simulink model "es2_sim2"  (R2023b)
settings: Solver=VariableStepAuto  StartTime=0.0  StopTime=10.0  RelTol=1e-3
values from neighbouring files (symbols this model uses):
  x0 = [3 5]'    [es2.m]    (also in es2_2.m = [3;5])
settings Model: Creator=stefa  LastModifiedBy=stefa

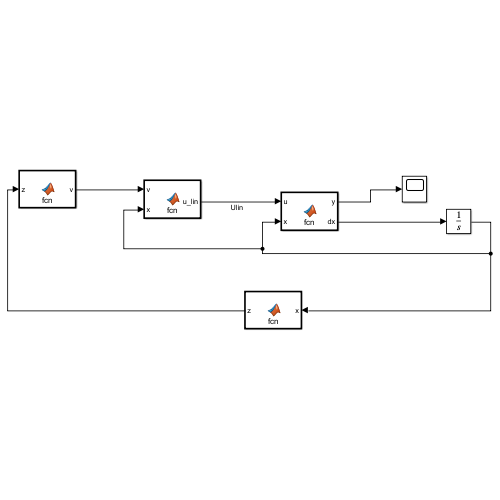
[thumbnail: Simulink's stored preview of the top-level diagram]
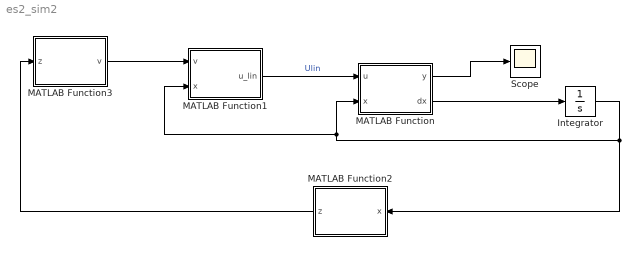
== system es2_sim2 ==
  Integrator : Integrator  InitialCondition=x0
  MATLAB Function : MATLAB Function  TreatAsAtomicUnit=on
  MATLAB Function1 : MATLAB Function  TreatAsAtomicUnit=on
  MATLAB Function2 : MATLAB Function  TreatAsAtomicUnit=on
  MATLAB Function3 : MATLAB Function  TreatAsAtomicUnit=on
  Scope : Scope
  wires:
  MATLAB Function/1(y) -> Scope/1
  MATLAB Function/2(dx) -> Integrator/1
  Integrator/1 -> MATLAB Function2/1(x), MATLAB Function1/2(x), MATLAB Function/2(x)
  MATLAB Function1/1(u_lin) -> MATLAB Function/1(u)  "Ulin"
  MATLAB Function3/1(v) -> MATLAB Function1/1(v)
  MATLAB Function2/1(z) -> MATLAB Function3/1(z)

== matlab function es2_sim2/MATLAB Function ==
  data: u input; y output; x input; dx output
function [y,dx]= fcn(u,x)
x1=x(1);
x2=x(2);

dx=[(x1^2+x1)*x2;-2*x2+x1-x2*u+6*u];

y=5*x1;

== matlab function es2_sim2/MATLAB Function2 ==
  data: x input; z output
function z = fcn(x)
x1=x(1);
x2=x(2);
z= [ 5*x1;5*x2*(x1^2 + x1)]

== matlab function es2_sim2/MATLAB Function3 ==
  data: z input; v output
function v = fcn(z)
z1=z(1);
z2=z(2);
K=[50 15];
v=-K(1)*z1-K(2)*z2;

== matlab function es2_sim2/MATLAB Function1 ==
  data: v input; u_lin output; x input
function u_lin = fcn(v,x)
x1=x(1);
x2=x(2);

u_lin=((5*x1^2 + 5*x1)*(x1 - 2*x2) - v + 5*x2^2*(2*x1 + 1)*(x1^2 + x1))/((5*x1^2 + 5*x1)*(x2 - 6));
